simulink model "Nivel_Concentracao_MA"  (R2020a)
settings: Solver=VariableStepAuto  StartTime=0.0  StopTime=10.0  RelTol=1e-3
libraries: cstblocks x4
settings Model: Creator=Avell  LastModifiedBy=Avell

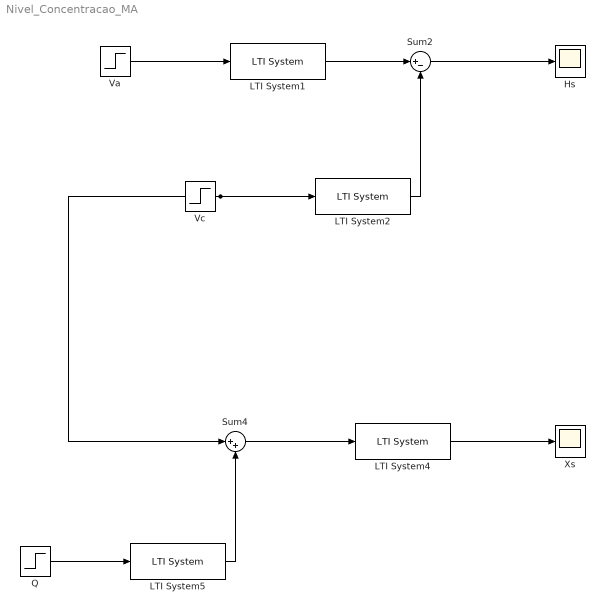
== system Nivel_Concentracao_MA ==
  Hs : Scope
  LTI System1 : cstblocks/LTI System  sys=Gh  IC=[]
  LTI System2 : cstblocks/LTI System  sys=Gvc  IC=[]
  LTI System4 : cstblocks/LTI System  sys=Gx  IC=[]
  LTI System5 : cstblocks/LTI System  sys=0.5  IC=[]
  Q : Step  Time=30  SampleTime=0
  Sum2 : Sum  Inputs=|+-
  Sum4 : Sum  Inputs=|++
  Va : Step  Time=30  SampleTime=0
  Vc : Step  Time=30  SampleTime=0
  Xs : Scope
  wires:
  LTI System1/1 -> Sum2/1
  Vc/1 -> LTI System2/1, Sum4/1
  Sum2/1 -> Hs/1
  LTI System2/1 -> Sum2/2
  Va/1 -> LTI System1/1
  LTI System4/1 -> Xs/1
  LTI System5/1 -> Sum4/2
  Sum4/1 -> LTI System4/1
  Q/1 -> LTI System5/1
